simulink model "l11"  (R2013a)
settings: Solver=ode45  StartTime=0.0  StopTime=30  RelTol=1e-3
libraries: simulink x1
settings Model: Creator=Sion  LastModifiedBy=Sion

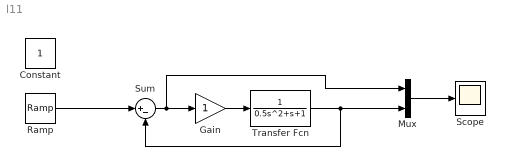
== system l11 ==
  Constant : Constant
  Gain : Gain
  Mux : Mux  Inputs=2
  Ramp : simulink/Sources/Ramp  slope=2  start=0  X0=0
  Scope : Scope
      settings: TimeRange=20  YMin=-2.41672e-62  YMax=10  SaveName=ScopeData5
  Sum : Sum  Inputs=|+-
  Transfer Fcn : TransferFcn  Denominator=[0.5 1 1]
  wires:
  Sum/1 -> Mux/1, Gain/1
  Gain/1 -> Transfer Fcn/1
  Transfer Fcn/1 -> Mux/2, Sum/2
  Ramp/1 -> Sum/1
  Mux/1 -> Scope/1
